simulink model "Torque_Vectoring_Controller_Controls_2018_Test"  (R2017b)
settings: Solver=ode45  StartTime=0.0  StopTime=inf  RelTol=1e-3  EnableMultiTasking=on
InitFcn:
  | clear_close
  | dataCar
  | optParam
  | structSensors
  | structSettings
  | structEstimPar
  | structAero
  | structVariables
  | readFuzzyFile
StartFcn:
  | clear_close
  | dataCar
  | optParam
  | structSensors
  | structSettings
  | structEstimPar
  | structAero
  | structVariables
  | readFuzzyFile
undefined symbols (not defined in the file or in its folder): car, sensors
libraries: CarMaker4SL x21, simulink x11
(part 4 of 4)

== matlab function Torque_Vectoring_Controller_Controls_2018_Test/CarMaker/Controls/Tire model//friction coefficient estimation/friction frank test   ==
  data: mu output; estimPar input; Magic_tire_param input; Fzi input; slip_ratio input; alpha_wheels input; States_matrix_front input
function mu  = frictionfrank(estimPar,Magic_tire_param,Fzi,slip_ratio, alpha_wheels, States_matrix_front)
%This function calculates an estimate for the maximum friction coefficient
%by comparing the estimated forces with the forces calculated using the
%Dugoff tire model for a certain side slip angle and slip ratio. The forces
%are calculated for a range of mu values, and the mu for which the forces
%deviate the least (rms) is chosen as the instantaneous mu value.
if length(States_matrix_front) >= 1000
    mu = [0.05;0.05;0.05;0.05];
    rms1 = [0;0;0;0];
    rms2 = [0;0;0;0];

    alpha_mu = [alpha_wheels.fl, alpha_wheels.fr, alpha_wheels.rl, alpha_wheels.rr];

    p0x = [Magic_tire_param.front_x; Magic_tire_param.front_x; ...
    Magic_tire_param.rear_x;Magic_tire_param.rear_x];
    p0y = [Magic_tire_param.front_y; Magic_tire_param.front_y; ...
        Magic_tire_param.rear_y;Magic_tire_param.rear_y];

    for i=1:1:4
        F_xd = Fzi(i)*p0x(i,3)*sin(p0x(i,2)*atan(p0x(i,1)*(1-p0x(i,4))*slip_ratio(i) + ...
            atan(p0x(i,1)*slip_ratio(i))));
        F_yd = Fzi(i)*p0y(i,3)*sin(p0y(i,2)*atan(p0y(i,1)*(1-p0y(i,4))*alpha_mu(i) + ...
            atan(p0y(i,1)*alpha_mu(i))));
   
        rms1(i) = sqrt((estimPar.Fxi(i)-F_xd)^2+(estimPar.Fyi(i)-F_yd)^2);
    end
    for i=1:1:4
        for mu1=0.1:0.05:1
            F_xd1 = Fzi(i)*p0x(i,3)*sin(p0x(i,2)*atan(p0x(i,1)*(1-p0x(i,4))*slip_ratio(i) + ...
                atan(p0x(i,1)*slip_ratio(i))));
            F_yd1 = Fzi(i)*p0y(i,3)*sin(p0y(i,2)*atan(p0y(i,1)*(1-p0y(i,4))*alpha_mu(i) + ...
                atan(p0y(i,1)*alpha_mu(i))));
            rms2(i) = sqrt((estimPar.Fxi(i)-F_xd1)^2+(estimPar.Fyi(i)-F_yd1)^2);
            if rms2(i) < rms1(i)
                mu(i) = mu1;
                rms1(i) = rms2(i);
            end
        end
    
    end
end

end

== matlab function Torque_Vectoring_Controller_Controls_2018_Test/CarMaker/Controls/Tire model//friction coefficient estimation/Magic tire param workspace ==
  data: Magic_tire_param input; Magic_Tire_Param_front_x output; Magic_Tire_Param_front_y output; Magic_Tire_Param_rear_x output; Magic_Tire_Param_rear_y output
function [Magic_Tire_Param_front_x, Magic_Tire_Param_front_y, Magic_Tire_Param_rear_x,...
    Magic_Tire_Param_rear_y] = MTF_workspace(Magic_tire_param)

Magic_Tire_Param_front_x = Magic_tire_param.front_x;
Magic_Tire_Param_front_y = Magic_tire_param.front_y;
Magic_Tire_Param_rear_x = Magic_tire_param.rear_x;
Magic_Tire_Param_rear_y = Magic_tire_param.rear_y;

end
